simulink model "compilation"  (Simulink 6.5)
settings: Solver=ode4  StartTime=0.0  StopTime=inf  FixedStep=0.001  RelTol=1e-3
libraries: opal_lib x4, rtlab x2, simulink x1
Description:
  | Model of a simple control system for use iin training.
settings Model: Creator=Paul Baracos  LastModifiedBy=BiaoYu
settings DataIOCC: SaveOutput=off  SaveTime=off  SignalLoggingName=sigsOut
settings OptimizationCC: BlockReduction=off  BooleanDataType=off  InlineInvariantSignals=on
settings DebuggingCC: SolverPrmCheckMsg=none  MultiTaskDSMMsg=warning  MultiTaskCondExecSysMsg=none  StrictBusMsg=None
settings HardwareCC: TargetUnknown=on
settings RTWCC: IncludeERTFirstTime=on

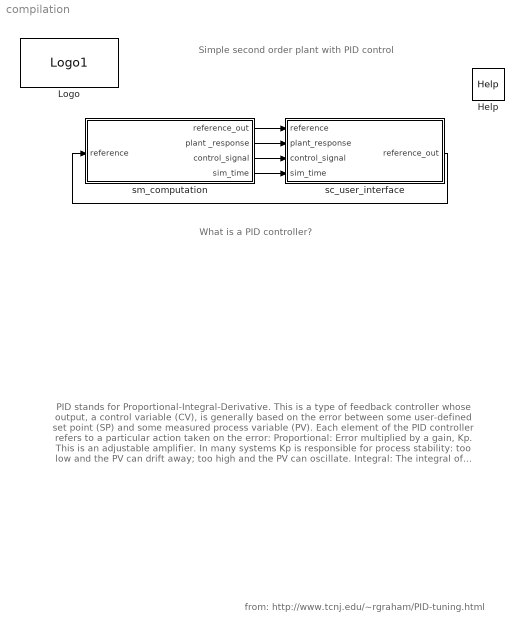
== system compilation ==
  note: Simple second order plant with PID control
  note: PID stands for Proportional-Integral-Derivative. This is a type of feedback controller whose output,
      | a control variable (CV), is generally based on the error between some user-defined set point
      | (SP) and some measured process variable (PV). Each element of the PID controller refers to a
      | particular action taken on the error:
      |
      | Proportional:
      | Error multiplied by a gain, Kp. This is an adjustable amplifier. In many systems Kp is
      | responsible for process stability: too low and the PV can drift away; too high and the
      | PV can oscillate.
      |
      | Integral:
      | The integral of error multiplied by a gain, Ki. In many systems Ki is responsible for
      | driving error to zero, but to set Ki too high is to invite oscillation or instability or
      | integrator windup or actuator saturation.
      |
      | Derivative:
      | The rate of change of error multiplied by a gain, Kd. In many systems Kd is responsible
      | for system response: too low and the PV will oscillate; too high and the PV will respond
      | sluggishly. The designer should also note that derivative action amplifies any noise in
      | the error signal.
      |
      | Tuning of a PID involves the adjustment of Kp, Ki, and Kd to achieve some user-defined
      | "optimal" character of system response.
      |
      | Although many architectures exist for control systems, the PID controller is mature and
      | well-understood by practitioners. For these reasons, it is often the first choice for new
      | controller design. It satisfies Occam's Razor in being the simplest solution for most cases.
  note: from: http://www.tcnj.edu/~rgraham/PID-tuning.html
  note: What is a PID controller?
  Help : opal_lib/Help  SystemSampleTime=-1  docfile=../../help/help_compilation.html
  Logo : opal_lib/Logo1  SystemSampleTime=-1
  sc_user_interface : Subsystem
  sm_computation : Subsystem
  wires:
  sc_user_interface/1(reference_out) -> sm_computation/1(reference)
  sm_computation/3(control_signal) -> sc_user_interface/3(control_signal)
  sm_computation/2(plant _response) -> sc_user_interface/2(plant_response)
  sm_computation/1(reference_out) -> sc_user_interface/1(reference)
  sm_computation/4(sim_time) -> sc_user_interface/4(sim_time)

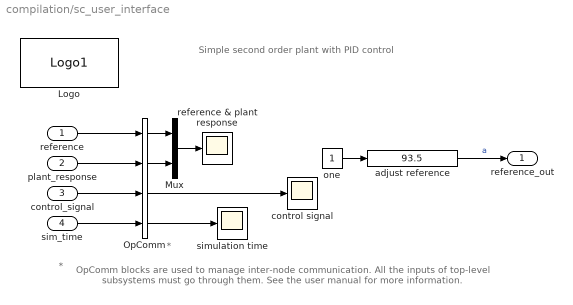
== system compilation/sc_user_interface ==
  note: Simple second order plant with PID control
  note: OpComm blocks are used to manage inter-node communication. All the inputs of top-level
      | subsystems must go through them. See the user manual for more information.
  note: *
  note: *
  reference : Inport
  plant_response : Inport  Port=2
  control_signal : Inport  Port=3
  sim_time : Inport  Port=4
  Logo : opal_lib/Logo1  SystemSampleTime=-1
  Mux : Mux  Inputs=2
  OpComm : rtlab/OpComm  SystemSampleTime=-1  nbport=4  groupe_acq=1  subsys_rate=0  st=0  Synchronization=on  Interpolation=on  Threshold=1.0  Missed_Data=off  Sim_Time=off  Samples=off  dynSigOut=off  from_console=0  warning_done=off  writeOpCommFile=off  Offset=off
  adjust reference : simulink/Math Operations/Slider Gain  SystemSampleTime=-1  low=0  gain=93.5  high=100
  control signal : Scope
      settings: YMin=-200  YMax=200  SaveName=controlSignal
  one : Constant  Value=1  OutDataType=sfix(16)  ConRadixGroup=Use specified scaling  OutScaling=2^0  SampleTime=inf  FramePeriod=inf
  reference & plant response : Scope
      settings: Tag=op_tm_save_it  TimeRange=10  YMin=0  YMax=160  SaveName=referenceAndPlant
  simulation time : Scope
      settings: YMin=-200  YMax=200  SaveName=controlSignal1
  reference_out : Outport
  wires:
  Mux/1 -> reference & plant response/1
  reference/1 -> OpComm/1
  control_signal/1 -> OpComm/3
  plant_response/1 -> OpComm/2
  OpComm/1 -> Mux/1
  OpComm/2 -> Mux/2
  OpComm/3 -> control signal/1
  adjust reference/1 -> reference_out/1  "a"
  one/1 -> adjust reference/1
  sim_time/1 -> OpComm/4
  OpComm/4 -> simulation time/1

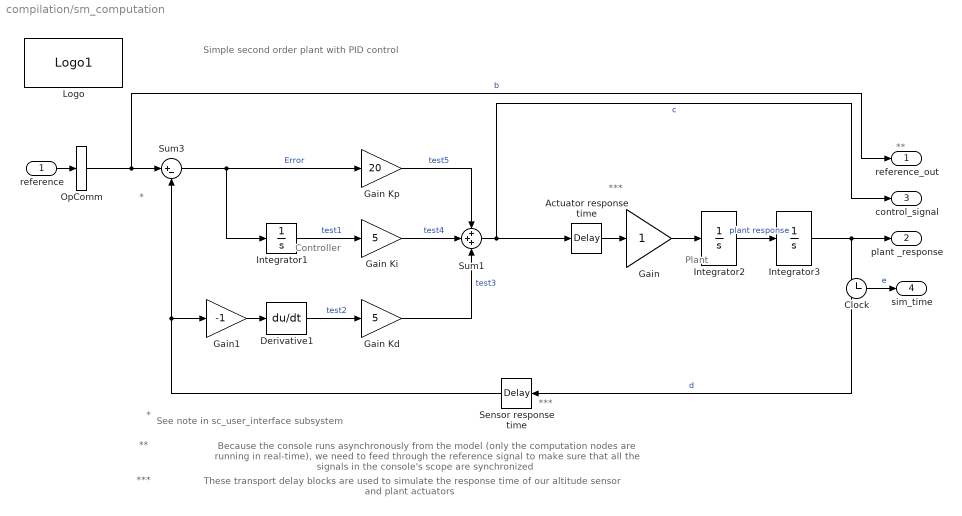
== system compilation/sm_computation ==
  note: Controller
  note: Plant
  note: Simple second order plant with PID control
  note: Because the console runs asynchronously from the model (only the computation nodes are running in real-time), we
      | need to feed through the reference signal to make sure that all the signals in the console's scope are synchronized
  note: **
  note: **
  note: *
  note: See note in sc_user_interface subsystem
  note: *
  note: ***
  note: These transport delay blocks are used to simulate the response time of our altitude sensor and plant actuators
  note: ***
  note: ***
  reference : Inport
  Actuator response time : TransportDelay  DelayTime=0.005
  Clock : Clock
      settings: Decimation=10
  Derivative1 : Derivative
  Gain : Gain  SaturateOnIntegerOverflow=on
  Gain Kd : Gain  Gain=5  SaturateOnIntegerOverflow=on
  Gain Ki : Gain  Gain=5  SaturateOnIntegerOverflow=on
  Gain Kp : Gain  Gain=20  SaturateOnIntegerOverflow=on
  Gain1 : Gain  Gain=-1  SaturateOnIntegerOverflow=on
  Integrator1 : Integrator
  Integrator2 : Integrator
  Integrator3 : Integrator  LimitOutput=on  UpperSaturationLimit=200  LowerSaturationLimit=0
  Logo : opal_lib/Logo1  SystemSampleTime=-1
  OpComm : rtlab/OpComm  SystemSampleTime=-1  nbport=1  groupe_acq=1  subsys_rate=0  st=0  Synchronization=on  Interpolation=on  Threshold=1.0  Missed_Data=off  Sim_Time=off  Samples=off  dynSigOut=off  from_console=0  warning_done=off  writeOpCommFile=off  Offset=off
  Sensor response time : TransportDelay  Orientation=left  DelayTime=0.005
  Sum1 : Sum  Inputs=+++  SaturateOnIntegerOverflow=on  InputSameDT=on
  Sum3 : Sum  Inputs=|+-  SaturateOnIntegerOverflow=on  InputSameDT=on
  reference_out : Outport
  plant _response : Outport  Port=2
  control_signal : Outport  Port=3
  sim_time : Outport  Port=4
  wires:
  reference/1 -> OpComm/1
  OpComm/1 -> Sum3/1, reference_out/1  "b"
  Sum3/1 -> Gain Kp/1, Integrator1/1  "Error"
  Gain Kp/1 -> Sum1/1  "test5"
  Integrator1/1 -> Gain Ki/1  "test1"
  Derivative1/1 -> Gain Kd/1  "test2"
  Gain Ki/1 -> Sum1/2  "test4"
  Gain1/1 -> Derivative1/1
  Gain Kd/1 -> Sum1/3  "test3"
  Sum1/1 -> control_signal/1, Actuator response time/1  "c"
  Sensor response time/1 -> Sum3/2, Gain1/1
  Integrator2/1 -> Integrator3/1  "plant response"
  Integrator3/1 -> plant _response/1, Sensor response time/1  "d"
  Gain/1 -> Integrator2/1
  Actuator response time/1 -> Gain/1
  Clock/1 -> sim_time/1  "e"
